simulink model "rotation"  (R2019a)
settings: Solver=VariableStepAuto  StartTime=0.0  StopTime=tf  FixedStep=100  RelTol=1e-3
InitFcn:
  | data
values from neighbouring files (symbols this model uses):
  inc = a    [data.m]
  inertia = [0.035, 0., 0.; 0., 0.02, 0.; 0., 0., 0.05]    [data.m]
  omega_d = omega_i    [data.m]
  raan = 52    [block_environment.m]    (also in data.m = b)
libraries: blocklib x5, vrlib x1
settings Model: Creator=imanol  LastModifiedBy=Imanol
settings DataIOCC: ReturnWorkspaceOutputs=off
settings DebuggingCC: ArithmeticOperatorsInVariantConditions=warning

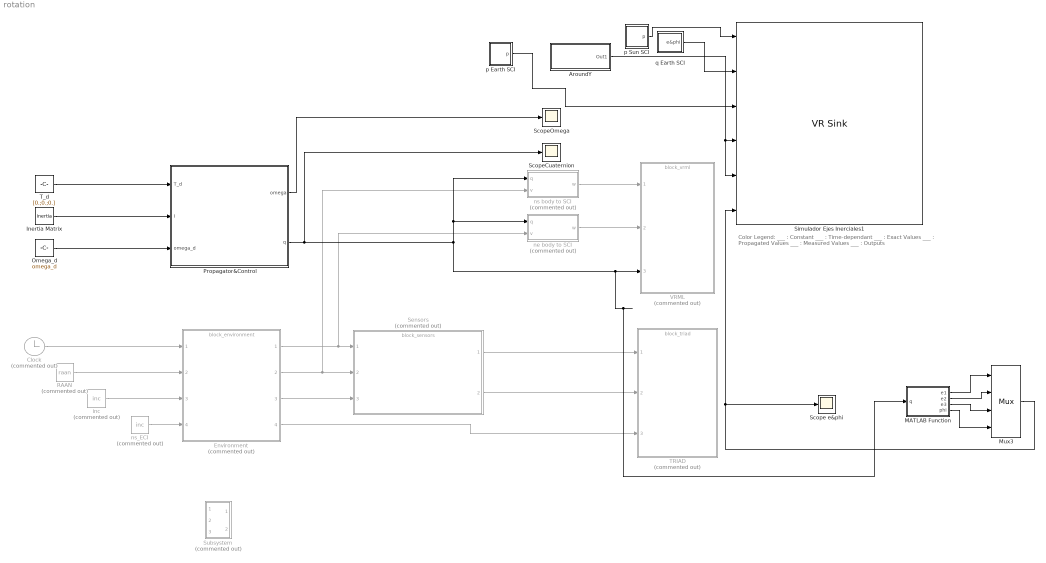
== system rotation ==
  note: Color Legend:
      | ___ : Constant
      | ___ : Time-dependant
      | ___ : Exact Values
      | ___ : Propagated Values
      | ___ : Measured Values
      | ___ : Outputs
  AroundY : Subsystem
  Clock : Clock  Commented=on
  Environment : ModelReference  Commented=on  ModelNameDialog=block_environment  SimulationMode=Normal  ModelReferenceVersion=1.3
  Inertia Matrix : Constant  Value=inertia
  MATLAB Function : MATLAB Function  TreatAsAtomicUnit=on
  Mux3 : Mux
  Omega_d : Constant  Value=omega_d
  Propagator&Control : Subsystem
  RAAN : Constant  Commented=on  Value=raan
  Scope e&phi : Scope
  ScopeCuaternion : Scope
  ScopeOmega : Scope
  Sensors : ModelReference  Commented=on  ModelNameDialog=block_sensors  SimulationMode=Normal  ModelReferenceVersion=1.4
  Simulador Ejes Inerciales1 : vrlib/VR Sink  InstantiateOnLoad=on  SampleTime=1e-2  ViewEnable=on  RemoteChange=off  RemoteView=off  FieldsWritten=StarSun.translation.3.1.1.double#PlanetEarth.rotation.4.1.1.double#PlanetEarth.translation.3.1.1.double#BillSun.rotation.4.1.1.double#BillEarth.rotation.4.1.1.double#BodyCoor.rotation.4.1.1.double  WorldFileName=vrml_mainV5.wrl  WorldDescription=Super Cubas World 2  AutoView=off  VideoDimensions=[]  AllowVariableSize=off
      settings: SourceProductBaseCode=VR
  Subsystem : Subsystem  Commented=on
  TRIAD : ModelReference  Commented=on  ModelNameDialog=block_triad  SimulationMode=Normal  ModelReferenceVersion=1.2
  T_d : Constant  Value=[0.;0.;0.]
  VRML : ModelReference  Commented=on  ModelNameDialog=block_vrml  SimulationMode=Normal  ModelReferenceVersion=1.17
  inc : Constant  Commented=on  Value=inc
  ne body to SCI : Subsystem  Commented=on
  ns body to SCI : Subsystem  Commented=on
  ns_ECI : Constant  Commented=on  Value=inc
  p Earth SCI : Subsystem
  p Sun SCI : Subsystem
  q Earth SCI : Subsystem
  wires:
  Environment/4 -> TRIAD/3
  Clock/1 -> Environment/1
  RAAN/1 -> Environment/2
  inc/1 -> Environment/3
  ns_ECI/1 -> Environment/4
  Environment/2 -> Sensors/2, ns body to SCI/2(v)
  Environment/3 -> Sensors/3
  Sensors/1 -> TRIAD/1
  Sensors/2 -> TRIAD/2
  ns body to SCI/1(w) -> VRML/1
  ne body to SCI/1(w) -> VRML/2
  Environment/1 -> ne body to SCI/2(v), Sensors/1
  T_d/1 -> Propagator&Control/1(T_d)
  Inertia Matrix/1 -> Propagator&Control/2(I)
  Omega_d/1 -> Propagator&Control/3(omega_d)
  Propagator&Control/1(omega) -> ScopeOmega/1
  AroundY/1(Out1) -> Simulador Ejes Inerciales1/4, Simulador Ejes Inerciales1/5
  p Earth SCI/1(p) -> Simulador Ejes Inerciales1/3
  q Earth SCI/1(e&phi) -> Simulador Ejes Inerciales1/2
  p Sun SCI/1(p) -> Simulador Ejes Inerciales1/1
  Mux3/1 -> Simulador Ejes Inerciales1/6, Scope e&phi/1
  Propagator&Control/2(q) -> ScopeCuaternion/1, ns body to SCI/1(q), ne body to SCI/1(q), MATLAB Function/1(q), VRML/3
  MATLAB Function/3(e3) -> Mux3/3
  MATLAB Function/1(e1) -> Mux3/1
  MATLAB Function/2(e2) -> Mux3/2
  MATLAB Function/4(phi) -> Mux3/4

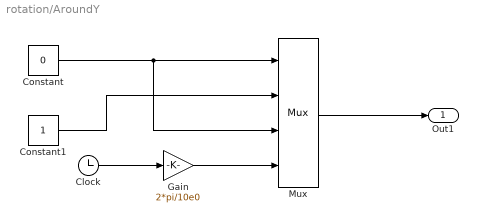
== system rotation/AroundY ==
  Clock : Clock
  Constant : Constant  Value=0
  Constant1 : Constant
  Gain : Gain  Gain=2*pi/10e0
  Mux : Mux
  Out1 : Outport
  wires:
  Clock/1 -> Gain/1
  Mux/1 -> Out1/1
  Gain/1 -> Mux/4
  Constant/1 -> Mux/3, Mux/1
  Constant1/1 -> Mux/2

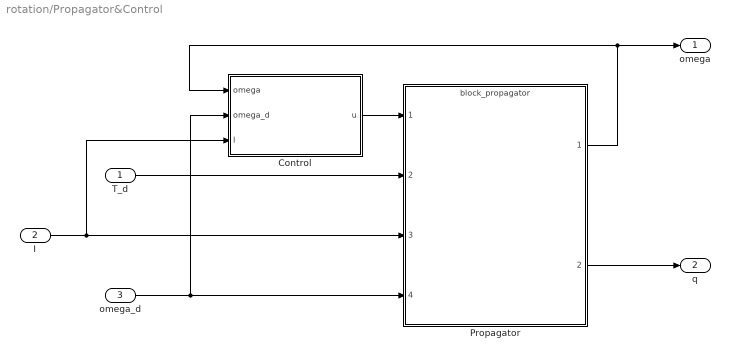
== system rotation/Propagator&Control ==
  T_d : Inport
  I : Inport  Port=2
  omega_d : Inport  Port=3
  Control : Subsystem
  Propagator : ModelReference  ModelNameDialog=block_propagator  SimulationMode=Normal  ModelReferenceVersion=1.8
  omega : Outport
  q : Outport  Port=2
  wires:
  I/1 -> Control/3(I), Propagator/3
  T_d/1 -> Propagator/2
  omega_d/1 -> Control/2(omega_d), Propagator/4
  Propagator/1 -> omega/1, Control/1(omega)
  Control/1(u) -> Propagator/1
  Propagator/2 -> q/1

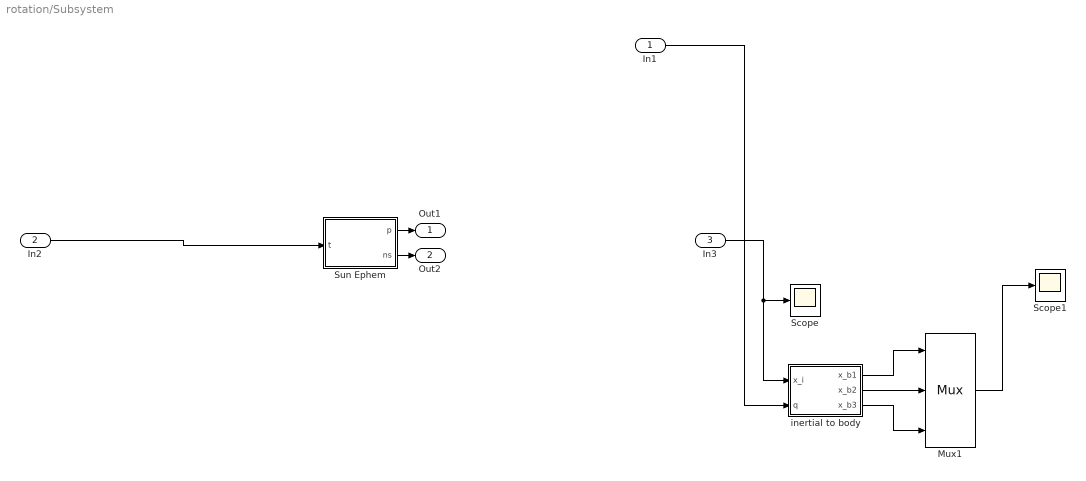
== system rotation/Subsystem ==
  In1 : Inport
  In2 : Inport  Port=2
  In3 : Inport  Port=3
  Mux1 : Mux  Inputs=3
  Scope : Scope
  Scope1 : Scope
  Sun Ephem : MATLAB Function  TreatAsAtomicUnit=on
  inertial to body : MATLAB Function  TreatAsAtomicUnit=on
  Out1 : Outport
  Out2 : Outport  Port=2
  wires:
  Sun Ephem/1(p) -> Out1/1
  In3/1 -> inertial to body/1(x_i), Scope/1
  In1/1 -> inertial to body/2(q)
  Mux1/1 -> Scope1/1
  Sun Ephem/2(ns) -> Out2/1
  inertial to body/3(x_b3) -> Mux1/3
  inertial to body/1(x_b1) -> Mux1/1
  inertial to body/2(x_b2) -> Mux1/2
  In2/1 -> Sun Ephem/1(t)

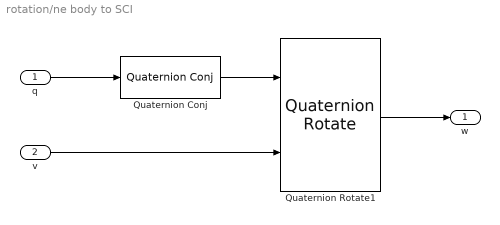
== system rotation/ne body to SCI ==
  q : Inport
  v : Inport  Port=2
  Quaternion Conj : blocklib/Quaternion Conj  SystemSampleTime=-1
      settings: SourceProductName=Custom Library
  Quaternion Rotate1 : blocklib/Quaternion Rotate  SystemSampleTime=-1
      settings: SourceProductName=Custom Library
  w : Outport
  wires:
  q/1 -> Quaternion Conj/1
  Quaternion Conj/1 -> Quaternion Rotate1/1
  v/1 -> Quaternion Rotate1/2
  Quaternion Rotate1/1 -> w/1

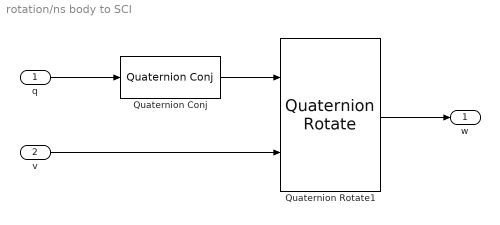
== system rotation/ns body to SCI ==
  q : Inport
  v : Inport  Port=2
  Quaternion Conj : blocklib/Quaternion Conj  SystemSampleTime=-1
      settings: SourceProductName=Custom Library
  Quaternion Rotate1 : blocklib/Quaternion Rotate  SystemSampleTime=-1
      settings: SourceProductName=Custom Library
  w : Outport
  wires:
  q/1 -> Quaternion Conj/1
  Quaternion Conj/1 -> Quaternion Rotate1/1
  v/1 -> Quaternion Rotate1/2
  Quaternion Rotate1/1 -> w/1

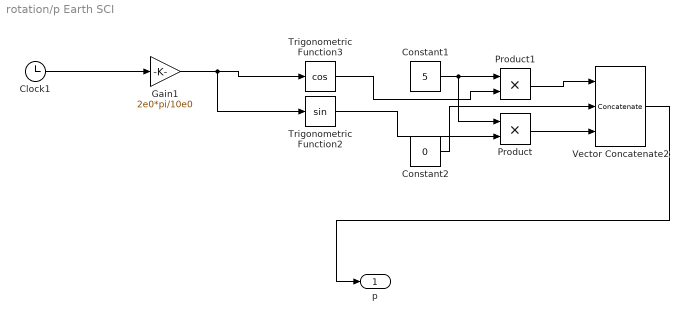
== system rotation/p Earth SCI ==
  Clock1 : Clock
  Constant1 : Constant  Value=5
  Constant2 : Constant  Value=0
  Gain1 : Gain  Gain=2e0*pi/10e0
  Product : Product
  Product1 : Product
  Trigonometric Function2 : Trigonometry
  Trigonometric Function3 : Trigonometry  Operator=cos
  Vector Concatenate2 : Concatenate  NumInputs=3
  p : Outport
  wires:
  Constant1/1 -> Product/1, Product1/1
  Trigonometric Function3/1 -> Product1/2
  Product/1 -> Vector Concatenate2/3
  Trigonometric Function2/1 -> Product/2
  Product1/1 -> Vector Concatenate2/1
  Constant2/1 -> Vector Concatenate2/2
  Clock1/1 -> Gain1/1
  Gain1/1 -> Trigonometric Function2/1, Trigonometric Function3/1
  Vector Concatenate2/1 -> p/1

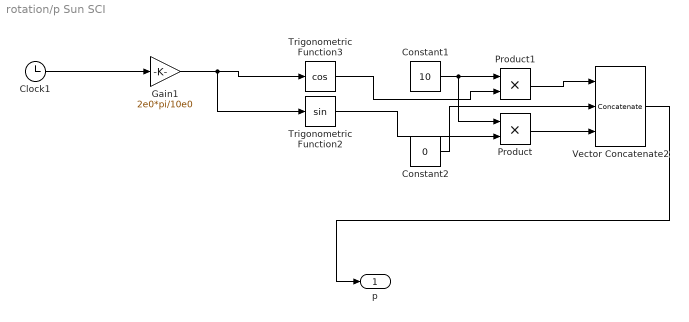
== system rotation/p Sun SCI ==
  Clock1 : Clock
  Constant1 : Constant  Value=10
  Constant2 : Constant  Value=0
  Gain1 : Gain  Gain=2e0*pi/10e0
  Product : Product
  Product1 : Product
  Trigonometric Function2 : Trigonometry
  Trigonometric Function3 : Trigonometry  Operator=cos
  Vector Concatenate2 : Concatenate  NumInputs=3
  p : Outport
  wires:
  Constant1/1 -> Product/1, Product1/1
  Trigonometric Function3/1 -> Product1/2
  Product/1 -> Vector Concatenate2/3
  Trigonometric Function2/1 -> Product/2
  Product1/1 -> Vector Concatenate2/1
  Constant2/1 -> Vector Concatenate2/2
  Clock1/1 -> Gain1/1
  Gain1/1 -> Trigonometric Function2/1, Trigonometric Function3/1
  Vector Concatenate2/1 -> p/1

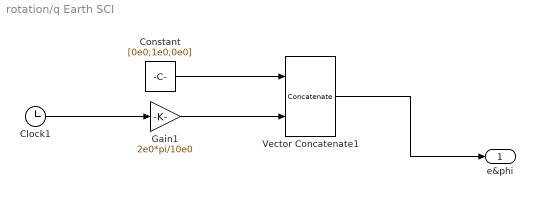
== system rotation/q Earth SCI ==
  Clock1 : Clock
  Constant : Constant  Value=[0e0;1e0;0e0]
  Gain1 : Gain  Gain=2e0*pi/10e0
  Vector Concatenate1 : Concatenate
  e&phi : Outport
  wires:
  Constant/1 -> Vector Concatenate1/1
  Clock1/1 -> Gain1/1
  Gain1/1 -> Vector Concatenate1/2
  Vector Concatenate1/1 -> e&phi/1

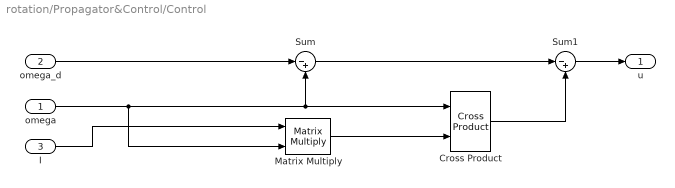
== system rotation/Propagator&Control/Control ==
  omega : Inport
  omega_d : Inport  Port=2
  I : Inport  Port=3
  Cross Product : blocklib/Cross Product  SystemSampleTime=-1
      settings: SourceProductName=Custom Library
  Matrix Multiply : Product  Multiplication=Matrix(*)
  Sum : Sum  Inputs=|-+
  Sum1 : Sum  Inputs=|-+
  u : Outport
  wires:
  omega/1 -> Matrix Multiply/2, Sum/2, Cross Product/1
  Matrix Multiply/1 -> Cross Product/2
  Sum/1 -> Sum1/1
  Sum1/1 -> u/1
  Cross Product/1 -> Sum1/2
  omega_d/1 -> Sum/1
  I/1 -> Matrix Multiply/1

== matlab function rotation/MATLAB Function ==
  data: q input; e1 output; e2 output; e3 output; phi output
function [e1, e2, e3, phi] = fcn(q)
ee2 = zeros(3, 1);
ee2(1) = q(1);
ee2(2) = q(2);
ee2(3) = q(3);
c_half = q(4);
if abs(abs(c_half) - 1e0) < 1e-5
    phi = 2e0 * acos(c_half);
    e1 = 1e0;
    e2 = 0e0;
    e3 = 0e0;
else
    s2_half = dot(ee2, ee2);
    s_half = sqrt(s2_half);
    phi = 2e0 * atan2d(s_half, c_half);
    e1 = ee2(1) / s_half;
    e2 = ee2(2) / s_half;
    e3 = ee2(3) / s_half;
end
% e = ee2 / norm(ee2);
% if (norm(e) < 1e-5)
%   phi = 0e0;
% else
%   if(abs(e(1)) > 1e-5)
%     s_half = ee2(1) / e(1);
%   elseif (abs(e(1)) > 1e-5)
%     s_half = ee2(2) / e(2);
%   else
%     s_half = ee2(3) / e(3);
%   end
%   phi = 2e0 * atan2(s_half, q(4));
% end
% %s = maxval(e2(abs(e2) > 1e-5) ./ e(abs(e2) > 1e-5));
% % phi = 2e0 * atan2(s, qq(4)) * 180. / pi;
% e1 = e(1);
% e2 = e(2);
% e3 = e(3);
% %phi = phi;
% 
% %q1 = qq(1);
% %q2 = qq(2);
% %q3 = qq(3);
% %q4 = qq(4);

== matlab function rotation/Subsystem/Sun Ephem ==
  data: t input; p output; ns output
function [p, ns] = fcn(t)
tf = 1e2;
inc = 98e0 * pi / 180e0;
nu = t / tf * 2e0 * pi * 12.0;
omega = t / tf * 2e0 * pi * 6.0;

c3 = [cos(-nu), sin(-nu), 0.; -sin(-nu), cos(-nu), 0.; 0., 0., 1.];
c1 = [1., 0., 0.; 0., cos(-inc), sin(-inc); 0., -sin(-inc), cos(-inc)];
c33 = [cos(-omega), sin(-omega), 0.; -sin(-omega), cos(-omega), 0.; 0., 0., 1.];

p = c33 * c1 * c3 * [200.; 0.; 0.];
ns = p / norm(p);

== matlab function rotation/Subsystem/inertial to body ==
  data: x_i input; x_b1 output; q input; x_b2 output; x_b3 output
function [x_b1, x_b2, x_b3] = fcn(x_i, q)

x_i_2 = zeros(4, 1);
x_i_2(1:3) = x_i;

q_ast = [-q(1); -q(2); -q(3); q(4)];

x_b_2 = q_mult(q, q_mult(x_i_2, q_ast));
x_b = x_b_2(1:3);
x_b1 = x_b(1);
x_b2 = x_b(2);
x_b3 = x_b(3);

function q3 = q_mult(q1, q2)
q3 = zeros(4,1);
q3(1:3) = q1(4) * q2(1:3) + q2(4) * q1(1:3) + cross(q1(1:3), q2(1:3));
q3(4) = q1(4) * q2(4) - dot(q1(1:3), q2(1:3));
